simulink model "matlabfun"  (R2025b)
settings: Solver=VariableStepAuto  StartTime=0.0  StopTime=10.0  RelTol=1e-3
undefined symbols (not defined in the file or in its folder): K_eig, x0_sylv
settings Model: Creator=salvo  LastModifiedBy=salvo

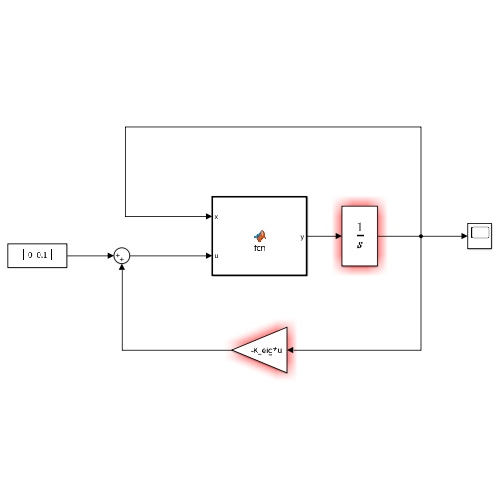
[thumbnail: Simulink's stored preview of the top-level diagram]
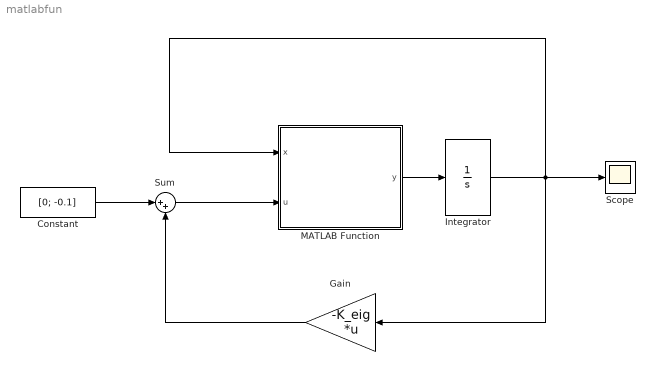
== system matlabfun ==
  Constant : Constant  Value=[0; -0.1]
  Gain : Gain  Gain=-K_eig  Multiplication=Matrix(K*u)
  Integrator : Integrator  InitialCondition=x0_sylv
  MATLAB Function : MATLAB Function  TreatAsAtomicUnit=on
  Scope : Scope
      settings: ActiveDisplayYMinimum=-0.19773157688819137  ActiveDisplayYMaximum=0.13308128632091015
  Sum : Sum  Inputs=|++
  wires:
  MATLAB Function/1(y) -> Integrator/1
  Integrator/1 -> MATLAB Function/1(x), Gain/1, Scope/1
  Constant/1 -> Sum/1
  Sum/1 -> MATLAB Function/2(u)
  Gain/1 -> Sum/2

== matlab function matlabfun/MATLAB Function ==
  data: x input; u input; y output
function y = fcn(x, u)
%#codegen

x1 = x(1);
x2 = x(2);
x3 = x(4);
x4 = x(4);



u1 = u(1);
u2 = u(2);


dx1 = x2;
dx2 = -0.8*sin(x1) - 0.5*x2 + 0.3*x4 +u1;
dx3 = x4;
dx4 = -0.6*sin(x3) - 0.4*x4 + 0.2*x2 + u2 + 0.1*cos(x1);



dxdt = [dx1;
        dx2;
        dx3;
        dx4];

y = dxdt;
